simulink subsystem "subsys_sphere_position"  (R2021a)
settings: Solver=VariableStepAuto  StartTime=0.0  StopTime=10.0  RelTol=1e-3
settings Model: Creator=antho  LastModifiedBy=antho

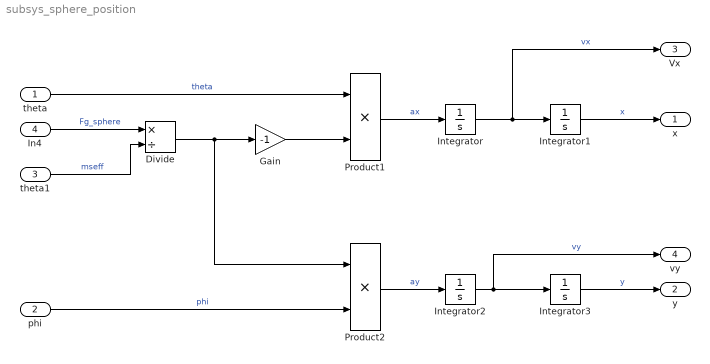
== system subsys_sphere_position ==
  theta : Inport
  phi : Inport  Port=2
  theta1 : Inport  Port=3
  In4 : Inport  Port=4
  Divide : Product  Inputs=*/
  Gain : Gain  Gain=-1
  Integrator{,1..3} (4 alike) : Integrator
  Product1 : Product
  Product2 : Product
  x : Outport
  y : Outport  Port=2
  Vx : Outport  Port=3
  vy : Outport  Port=4
  wires:
  theta/1 -> Product1/1  "theta"
  Integrator3/1 -> y/1  "y"
  phi/1 -> Product2/2  "phi"
  Product1/1 -> Integrator/1  "ax"
  Integrator1/1 -> x/1  "x"
  Integrator2/1 -> vy/1, Integrator3/1  "vy"
  Integrator/1 -> Integrator1/1, Vx/1  "vx"
  Product2/1 -> Integrator2/1  "ay"
  In4/1 -> Divide/1  "Fg_sphere"
  theta1/1 -> Divide/2  "mseff"
  Gain/1 -> Product1/2
  Divide/1 -> Gain/1, Product2/1
